simulink library "Digital"  (R2017a)
settings: Solver=VariableStepAuto  StartTime=0.0  StopTime=10.0  RelTol=1e-3
settings Model: Creator=Di Russo  LastModifiedBy=Vraj M

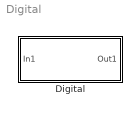
== system Digital ==
  Digital : Subsystem

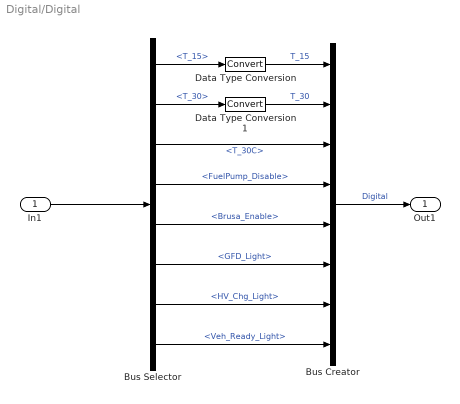
== system Digital/Digital ==
  In1 : Inport
  Bus Creator : BusCreator  Inputs=8
  Bus Selector : BusSelector  OutputSignals=BMS_Digital.T_15,BMS_Digital.T_30,BMS_Digital.T_30C,PUMP_Control.FuelPump_Disable,OBC_Digital.Brusa_Enable,Axiomatic_CAN.GFD_Light,Axiomatic_CAN.HV_Chg_Light,Axiomatic_CAN.Veh_Ready_Light
  Data Type Conversion : DataTypeConversion
  Data Type Conversion1 : DataTypeConversion
  Out1 : Outport
  wires:
  Data Type Conversion1/1 -> Bus Creator/2  "T_30"
  Data Type Conversion/1 -> Bus Creator/1  "T_15"
  Bus Selector/8 -> Bus Creator/8  "<Veh_Ready_Light>"
  Bus Selector/7 -> Bus Creator/7  "<HV_Chg_Light>"
  Bus Selector/6 -> Bus Creator/6  "<GFD_Light>"
  Bus Selector/5 -> Bus Creator/5  "<Brusa_Enable>"
  Bus Selector/1 -> Data Type Conversion/1  "<T_15>"
  Bus Selector/2 -> Data Type Conversion1/1  "<T_30>"
  Bus Selector/3 -> Bus Creator/3  "<T_30C>"
  Bus Selector/4 -> Bus Creator/4  "<FuelPump_Disable>"
  Bus Creator/1 -> Out1/1  "Digital"
  In1/1 -> Bus Selector/1
